simulink model "Pendulum_on_a_Cart"  (R2013b)
settings: Solver=ode3  SolverMode=SingleTasking  StartTime=0.0  StopTime=inf  RelTol=1e-3
values from neighbouring files (symbols this model uses):
  a_b = 0.8    [LEGO_PendulumOnCart_controller.m]    (also in matlab.mat)
  a_d = 0.8    [LEGO_PendulumOnCart_controller.m]    (also in matlab.mat)
  ts1 = 0.004    [LEGO Servo Motor experiments.mat]    (also in LEGO_PendulumOnCart_controller.m; matlab.mat)
  w_n = 172.3/(2*zeta)    (= 86.15)    [LEGO_PendulumOnCart_controller.m]    (also in matlab.mat = 7.59643879413)
  zeta = 1    [LEGO_PendulumOnCart_controller.m]    (also in matlab.mat)
undefined symbols (not defined in the file or in its folder): Kcp, Kv, sigbuilder_block
libraries: legonxtlib x12, simulink x1
settings Model: SimulationMode=external  ExtModeTrigDuration=2  Creator=Alphonso Monk  LastModifiedBy=Alphonso Monk
settings OptimizationCC: OptimizeModelRefInitCode=on  LifeSpan=1
settings DebuggingCC: SolverPrmCheckMsg=none
settings HardwareCC: ProdLargestAtomicInteger=Long  ProdLargestAtomicFloat=Float  ProdEndianess=LittleEndian  ProdHWDeviceType=ARM Compatible->ARM 7
settings RTWCC: SystemTargetFile=realtime.tlc  GenerateMakefile=off  TemplateMakefile=realtime.tmf  Description=Run on Target Hardware  RTWVerbose=off  ProcessScript=realtime_make_rtw_hook
settings STFCustomTargetCC: TargetLibSuffix=.a  GenerateSampleERTMain=on  ERTCustomFileBanners=on  SupportNonInlinedSFcns=off  SupportVariableSizeSignals=on  MATLABClassNameForMDSCustomization=Simulink.SoftwareTarget.ERTCustomization  GRTInterface=off  SystemTargetFile=realtime.tlc
settings ERTTargetCC: CodeReplacementLibrary=ANSI_C  GenerateSampleERTMain=on  ParMdlRefBuildCompliant=off  CompOptLevelCompliant=off  ConcurrentExecutionCompliant=off  CombineOutputUpdateFcns=off  ERTFirstTimeCompliant=off  SupportContinuousTime=on  SupportVariableSizeSignals=on  ModelStepFunctionPrototypeControlCompliant=off  CPPClassGenCompliant=off  ExtMode=on  ExtModeTransport=2  ExtModeMexFile=ext_serial_win32_comm_no_acks_rtt  ExtModeMexArgs=0 3 9600 30  InlinedParameterPlacement=NonHierarchical  ERTSrcFileBannerTemplate=realtime_code_template.cgt  ERTHdrFileBannerTemplate=realtime_code_template.cgt  ERTDataSrcFileTemplate=realtime_code_template.cgt  ERTDataHdrFileTemplate=realtime_code_template.cgt  ERTCustomFileTemplate=realtime_file_process.tlc

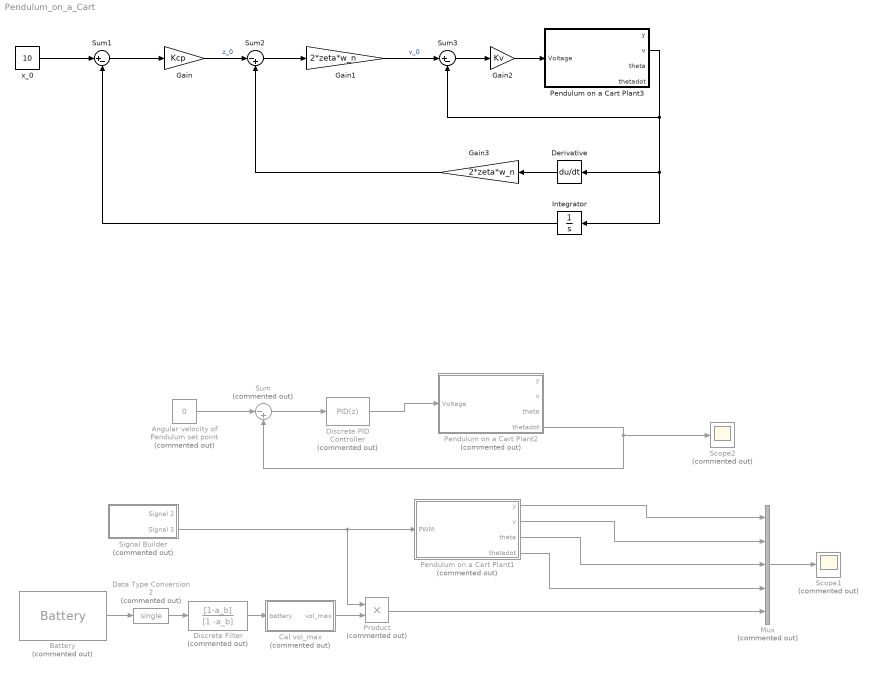
== system Pendulum_on_a_Cart ==
  Angular velocity of Pendulum set point : Constant  Commented=on  Value=0
  Battery : legonxtlib/Battery  Commented=on  sampleTime=ts1
  Cal vol_max : Subsystem  Commented=on
  Data Type Conversion2 : DataTypeConversion  Commented=on  OutDataTypeStr=single  RndMeth=Simplest
  Derivative : Derivative
  Discrete Filter : DiscreteFilter  Commented=on  Numerator=[1-a_b]  Denominator=[1 -a_b]
  Discrete PID Controller : simulink/Continuous/PID Controller  Commented=on  Controller=PID  TimeDomain=Discrete-time  SampleTime=ts1  IntegratorMethod=Forward Euler  FilterMethod=Forward Euler  Form=Parallel  P=0.4059  I=0  D=0  N=100  InitialConditionSource=internal  InitialConditionForIntegrator=0  InitialConditionForFilter=0  ExternalReset=none  LimitOutput=on  UpperSaturationLimit=9  LowerSaturationLimit=-9  LinearizeAsGain=off  AntiWindupMode=none  Kb=1  TrackingMode=off  Kt=1  PParamMin=[]  PParamMax=[]  IParamMin=[]  IParamMax=[]  DParamMin=[]  DParamMax=[]  NParamMin=[]  NParamMax=[]  KbParamMin=[]  KbParamMax=[]  KtParamMin=[]  KtParamMax=[]  POutMin=[]  POutMax=[]  IOutMin=[]  IOutMax=[]  DOutMin=[]  DOutMax=[]  NOutMin=[]  NOutMax=[]  KbOutMin=[]  KbOutMax=[]  KtOutMin=[]  KtOutMax=[]  IntegratorOutMin=[]  IntegratorOutMax=[]  FilterOutMin=[]  FilterOutMax=[]  SumOutMin=[]  SumOutMax=[]  SumI1OutMin=[]  SumI1OutMax=[]  SumI2OutMin=[]  SumI2OutMax=[]  SumI3OutMin=[]  SumI3OutMax=[]  SumDOutMin=[]  SumDOutMax=[]  SaturationOutMin=[]  SaturationOutMax=[]  IntegratorContinuousStateAttributes=''  IntegratorStateMustResolveToSignalObject=off  IntegratorRTWStateStorageClass=Auto  FilterContinuousStateAttributes=''  FilterStateMustResolveToSignalObject=off  FilterRTWStateStorageClass=Auto
  Gain : Gain  Gain=Kcp
  Gain1 : Gain  Gain=2*zeta*w_n
  Gain2 : Gain  Gain=Kv
  Gain3 : Gain  Gain=2*zeta*w_n
  Integrator : Integrator
  Mux : Mux  Commented=on  Inputs=5
  Pendulum on a Cart Plant1 : Subsystem  Commented=on
  Pendulum on a Cart Plant2 : Subsystem  Commented=on
  Pendulum on a Cart Plant3 : Subsystem
  Product : Product  Commented=on
  Scope1 : Scope  Commented=on
      settings: YMin=-600  YMax=600  SaveName=motorResponse1
  Scope2 : Scope  Commented=on
      settings: YMin=1026  YMax=1134  SaveName=motorResponse
  Signal Builder : Subsystem  Tag=STV Subsys  Commented=on  LoadFcn=sigbuilder_block('load');  StartFcn=sigbuilder_block('start');  StopFcn=sigbuilder_block('stop');  ClipboardFcn=sigbuilder_block('clipboard');  mask(Sigbuilder block){}
      mask help: Simulink:masks:SigbuilderBlock_MD
      mask init:
      | if ~strcmp(get_param(bdroot(gcbh),'SimulationStatus'),'stopped') tuvar = sigbuilder_block('maskInit'); end
      settings: CopyFcn=sigbuilder_block('copy');  DeleteFcn=sigbuilder_block('delete');  ModelCloseFcn=sigbuilder_block('modelClose');  PreSaveFcn=sigbuilder_block('preSave');  PauseFcn=sigbuilder_block('pause');  ContinueFcn=sigbuilder_block('continue');  NameChangeFcn=sigbuilder_block('namechange');  OpenFcn=sigbuilder_block('open',[6 28.5 1012.5 484.5 ]);  CloseFcn=sigbuilder_block('close');
      mask Display: plot(0, 0, 100, 100,[2, 2, 32, 32, 2], [68, 8, 8, 68, 68],[32, 2], [38, 38], [32, 19, 2],[53, 60, 44], [32, 17, 17, 2],[16, 16, 31, 31]);txt = getActiveGroup(gcbh);text(2, 100, txt,'verticalAlignment', 'top');
  Sum : Sum  Commented=on  Inputs=|-+
  Sum1 : Sum  Inputs=|+-
  Sum2 : Sum  Inputs=|-+
  Sum3 : Sum  Inputs=|+-
  x_0 : Constant  Value=10
  wires:
  Mux/1 -> Scope1/1
  Signal Builder/2(Signal 3) -> Product/1, Pendulum on a Cart Plant1/1(PWM)
  Product/1 -> Mux/5
  Discrete PID Controller/1 -> Pendulum on a Cart Plant2/1(Voltage)
  Pendulum on a Cart Plant2/4(thetadot) -> Scope2/1, Sum/2
  Sum/1 -> Discrete PID Controller/1
  Angular velocity of Pendulum set point/1 -> Sum/1
  Discrete Filter/1 -> Cal vol_max/1(battery)
  Data Type Conversion2/1 -> Discrete Filter/1
  Battery/1 -> Data Type Conversion2/1
  Cal vol_max/1(vol_max) -> Product/2
  Pendulum on a Cart Plant1/1(y) -> Mux/1
  Pendulum on a Cart Plant1/2(v) -> Mux/2
  Pendulum on a Cart Plant1/3(theta) -> Mux/3
  Pendulum on a Cart Plant1/4(thetadot) -> Mux/4
  x_0/1 -> Sum1/1
  Sum1/1 -> Gain/1
  Gain/1 -> Sum2/1  "z_0"
  Sum2/1 -> Gain1/1
  Gain1/1 -> Sum3/1  "v_0"
  Sum3/1 -> Gain2/1
  Gain2/1 -> Pendulum on a Cart Plant3/1(Voltage)
  Pendulum on a Cart Plant3/2(v) -> Integrator/1, Derivative/1, Sum3/2
  Derivative/1 -> Gain3/1
  Gain3/1 -> Sum2/2
  Integrator/1 -> Sum1/2

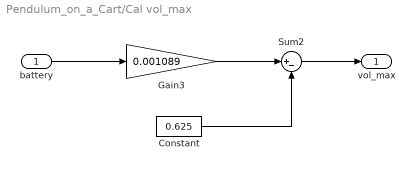
== system Pendulum_on_a_Cart/Cal vol_max ==
  battery : Inport
  Constant : Constant  Value=0.625  OutDataTypeStr=single
      settings: AttributesFormatString=DataType = %<OutDataTypeStr>
  Gain3 : Gain  Gain=0.001089  OutDataTypeStr=Inherit: Same as input  ParamDataTypeStr=Inherit: Same as input
  Sum2 : Sum  Inputs=|+-  OutDataTypeStr=Inherit: Same as first input
  vol_max : Outport
  wires:
  Gain3/1 -> Sum2/1
  Sum2/1 -> vol_max/1
  Constant/1 -> Sum2/2
  battery/1 -> Gain3/1

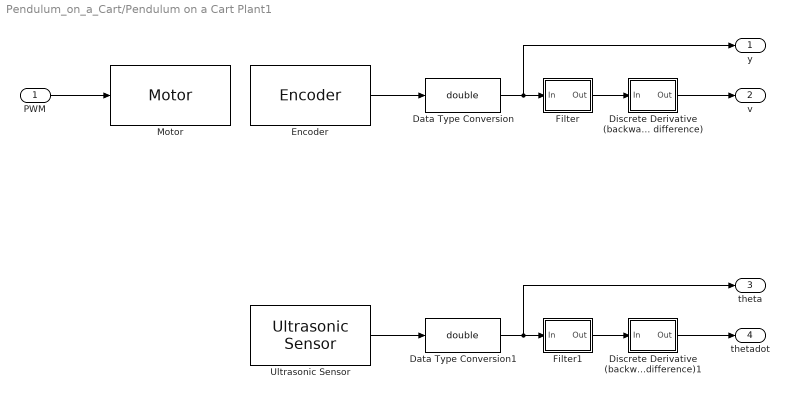
== system Pendulum_on_a_Cart/Pendulum on a Cart Plant1 ==
  PWM : Inport
  Data Type Conversion : DataTypeConversion  OutDataTypeStr=double
  Data Type Conversion1 : DataTypeConversion  OutDataTypeStr=double
  Discrete Derivative (backward difference) : Subsystem
  Discrete Derivative (backward difference)1 : Subsystem
  Encoder : legonxtlib/Encoder  portNumber=B  opMode=No reset  sampleTime=ts1
  Filter : Subsystem
  Filter1 : Subsystem
  Motor : legonxtlib/Motor  sportNumber=B  sstopAction=Brake
  Ultrasonic Sensor : legonxtlib/Ultrasonic Sensor  PortNumber=4  sampleTime=ts1
  y : Outport
  v : Outport  Port=2
  theta : Outport  Port=3
  thetadot : Outport  Port=4
  wires:
  Ultrasonic Sensor/1 -> Data Type Conversion1/1
  Data Type Conversion1/1 -> Filter1/1(In), theta/1
  Filter1/1(Out) -> Discrete Derivative (backward difference)1/1(In)
  Discrete Derivative (backward difference)1/1(Out) -> thetadot/1
  PWM/1 -> Motor/1
  Data Type Conversion/1 -> y/1, Filter/1(In)
  Filter/1(Out) -> Discrete Derivative (backward difference)/1(In)
  Discrete Derivative (backward difference)/1(Out) -> v/1
  Encoder/1 -> Data Type Conversion/1

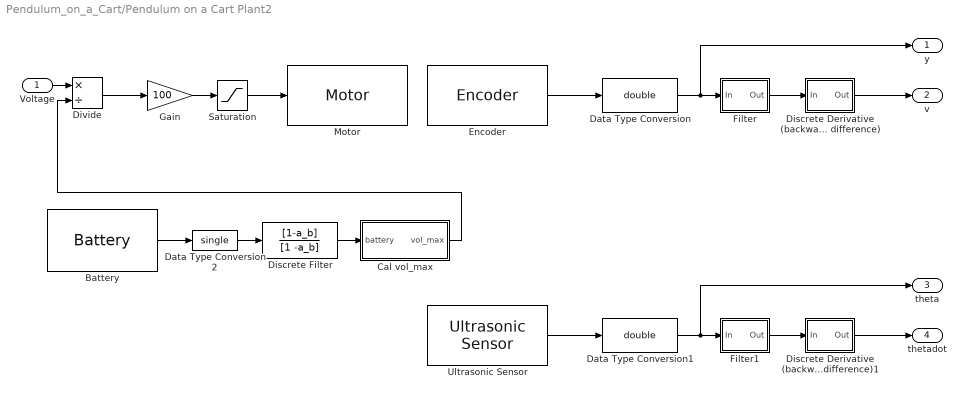
== system Pendulum_on_a_Cart/Pendulum on a Cart Plant2 ==
  Voltage : Inport
  Battery : legonxtlib/Battery  sampleTime=ts1
  Cal vol_max : Subsystem
  Data Type Conversion : DataTypeConversion  OutDataTypeStr=double
  Data Type Conversion1 : DataTypeConversion  OutDataTypeStr=double
  Data Type Conversion2 : DataTypeConversion  OutDataTypeStr=single  RndMeth=Simplest
  Discrete Derivative (backward difference) : Subsystem
  Discrete Derivative (backward difference)1 : Subsystem
  Discrete Filter : DiscreteFilter  Numerator=[1-a_b]  Denominator=[1 -a_b]
  Divide : Product  Inputs=*/
  Encoder : legonxtlib/Encoder  portNumber=B  opMode=No reset  sampleTime=ts1
  Filter : Subsystem
  Filter1 : Subsystem
  Gain : Gain  Gain=100
  Motor : legonxtlib/Motor  sportNumber=B  sstopAction=Brake
  Saturation : Saturate  UpperLimit=100  LowerLimit=-100
  Ultrasonic Sensor : legonxtlib/Ultrasonic Sensor  PortNumber=4  sampleTime=ts1
  y : Outport
  v : Outport  Port=2
  theta : Outport  Port=3
  thetadot : Outport  Port=4
  wires:
  Encoder/1 -> Data Type Conversion/1
  Discrete Derivative (backward difference)/1(Out) -> v/1
  Filter/1(Out) -> Discrete Derivative (backward difference)/1(In)
  Data Type Conversion/1 -> Filter/1(In), y/1
  Gain/1 -> Saturation/1
  Battery/1 -> Data Type Conversion2/1
  Data Type Conversion2/1 -> Discrete Filter/1
  Discrete Filter/1 -> Cal vol_max/1(battery)
  Voltage/1 -> Divide/1
  Cal vol_max/1(vol_max) -> Divide/2
  Divide/1 -> Gain/1
  Saturation/1 -> Motor/1
  Discrete Derivative (backward difference)1/1(Out) -> thetadot/1
  Filter1/1(Out) -> Discrete Derivative (backward difference)1/1(In)
  Data Type Conversion1/1 -> theta/1, Filter1/1(In)
  Ultrasonic Sensor/1 -> Data Type Conversion1/1

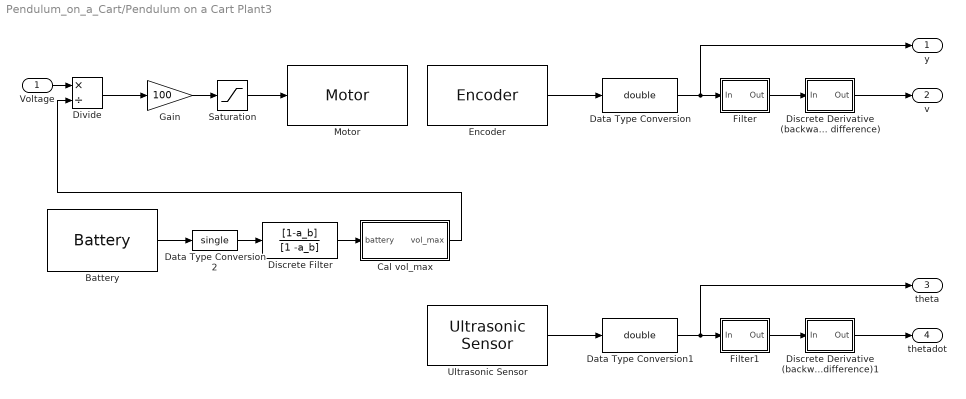
== system Pendulum_on_a_Cart/Pendulum on a Cart Plant3 ==
  Voltage : Inport
  Battery : legonxtlib/Battery  sampleTime=ts1
  Cal vol_max : Subsystem
  Data Type Conversion : DataTypeConversion  OutDataTypeStr=double
  Data Type Conversion1 : DataTypeConversion  OutDataTypeStr=double
  Data Type Conversion2 : DataTypeConversion  OutDataTypeStr=single  RndMeth=Simplest
  Discrete Derivative (backward difference) : Subsystem
  Discrete Derivative (backward difference)1 : Subsystem
  Discrete Filter : DiscreteFilter  Numerator=[1-a_b]  Denominator=[1 -a_b]
  Divide : Product  Inputs=*/
  Encoder : legonxtlib/Encoder  portNumber=B  opMode=No reset  sampleTime=ts1
  Filter : Subsystem
  Filter1 : Subsystem
  Gain : Gain  Gain=100
  Motor : legonxtlib/Motor  sportNumber=B  sstopAction=Brake
  Saturation : Saturate  UpperLimit=100  LowerLimit=-100
  Ultrasonic Sensor : legonxtlib/Ultrasonic Sensor  PortNumber=4  sampleTime=ts1
  y : Outport
  v : Outport  Port=2
  theta : Outport  Port=3
  thetadot : Outport  Port=4
  wires:
  Ultrasonic Sensor/1 -> Data Type Conversion1/1
  Data Type Conversion1/1 -> Filter1/1(In), theta/1
  Filter1/1(Out) -> Discrete Derivative (backward difference)1/1(In)
  Discrete Derivative (backward difference)1/1(Out) -> thetadot/1
  Saturation/1 -> Motor/1
  Divide/1 -> Gain/1
  Cal vol_max/1(vol_max) -> Divide/2
  Voltage/1 -> Divide/1
  Discrete Filter/1 -> Cal vol_max/1(battery)
  Data Type Conversion2/1 -> Discrete Filter/1
  Battery/1 -> Data Type Conversion2/1
  Gain/1 -> Saturation/1
  Data Type Conversion/1 -> y/1, Filter/1(In)
  Filter/1(Out) -> Discrete Derivative (backward difference)/1(In)
  Discrete Derivative (backward difference)/1(Out) -> v/1
  Encoder/1 -> Data Type Conversion/1

== system Pendulum_on_a_Cart/Signal Builder ==
  Demux : Demux  Tag=STV Demux  Outputs=2
  FromWs : FromWorkspace  Tag=STV FromWs  VariableName=tuvar  SampleTime=0
      SigBuilderData=|
      | common.afterFinalStr = 'Extrapolate'
      | common.sampleTime = 0
      | dataSet.timeRange = [0 30]
      | dataSet.name = 'Group 1'
      | sbobj.Groups.Name = 'Group 1'
      | sbobj.Groups.Signals(1).Name = 'Signal 2'
      | sbobj.Groups.Signals(1).XData = [0 3 3 7 7 30]
      | sbobj.Groups.Signals(1).YData = [0 0 100 100 0 0]
      | sbobj.Groups.Signals(2).Name = 'Signal 3'
      | sbobj.Groups.Signals(2).XData = [0 1 1 1.5 1.5 2.5 2.5 3.5 3.5 5 5 5.5 5.5 6.5 6.5 7 7 7.5 7.5 8.5 8.5 10.5 10.5 11 11 13.5 13.5 14 14 14.5 14.5 15 15 15.5 15.5 17.5 17.5 18.5 18.5 19 19 19.5 19.5 21 21 22 22 23.5 23.5 25 25 25.5 25.5 26.5 26.5 28 28 28.5 28.5 29 29 29.5 29.5 30]
      | sbobj.Groups.Signals(2).YData = [100 100 -100 -100 100 100 -100 -100 100 100 -100 -100 100 100 -100 -100 100 100 -100 -100 100 100 -100 -100 100 100 -100 -100 100 100 -100 -100 100 100 -100 -100 100 100 -100 -100 100 100 -100 -100 100 100 -100 -100 100 100 -100 -100 100 100 -100 -100 100 100 -100 -100 100 100 -100 -100]
      | sbobj.Groups.TimeRange = [0 30]
  Signal 2 : Outport  Tag=STV Outport
  Signal 3 : Outport  Tag=STV Outport  Port=2
  wires:
  FromWs/1 -> Demux/1
  Demux/1 -> Signal 2/1
  Demux/2 -> Signal 3/1

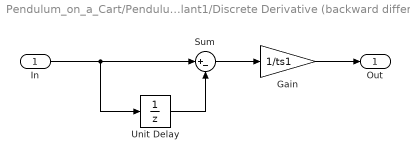
== system Pendulum_on_a_Cart/Pendulum on a Cart Plant1/Discrete Derivative (backward difference) ==
  In : Inport
  Gain : Gain  Gain=1/ts1  OutDataTypeStr=Inherit: Same as input  ParamDataTypeStr=Inherit: Same as input
  Sum : Sum  Inputs=|+-  OutDataTypeStr=Inherit: Same as first input
  Unit Delay : UnitDelay  SampleTime=-1
  Out : Outport
  wires:
  Sum/1 -> Gain/1
  Unit Delay/1 -> Sum/2
  In/1 -> Unit Delay/1, Sum/1
  Gain/1 -> Out/1

== system Pendulum_on_a_Cart/Pendulum on a Cart Plant1/Discrete Derivative (backward difference)1 ==
  In : Inport
  Gain : Gain  Gain=1/ts1  OutDataTypeStr=Inherit: Same as input  ParamDataTypeStr=Inherit: Same as input
  Sum : Sum  Inputs=|+-  OutDataTypeStr=Inherit: Same as first input
  Unit Delay : UnitDelay  SampleTime=-1
  Out : Outport
  wires:
  Gain/1 -> Out/1
  In/1 -> Sum/1, Unit Delay/1
  Unit Delay/1 -> Sum/2
  Sum/1 -> Gain/1

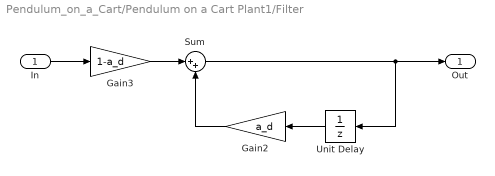
== system Pendulum_on_a_Cart/Pendulum on a Cart Plant1/Filter ==
  In : Inport
  Gain2 : Gain  Gain=a_d  OutDataTypeStr=Inherit: Same as input  ParamDataTypeStr=Inherit: Same as input
  Gain3 : Gain  Gain=1-a_d  OutDataTypeStr=Inherit: Same as input  ParamDataTypeStr=Inherit: Same as input
  Sum : Sum  Inputs=|++  OutDataTypeStr=Inherit: Same as first input
  Unit Delay : UnitDelay  SampleTime=-1
  Out : Outport
  wires:
  Sum/1 -> Unit Delay/1, Out/1
  Unit Delay/1 -> Gain2/1
  Gain2/1 -> Sum/2
  Gain3/1 -> Sum/1
  In/1 -> Gain3/1

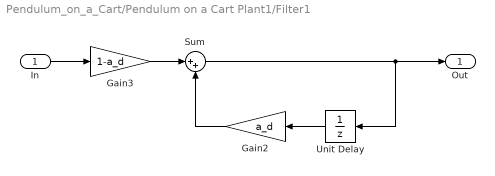
== system Pendulum_on_a_Cart/Pendulum on a Cart Plant1/Filter1 ==
  In : Inport
  Gain2 : Gain  Gain=a_d  OutDataTypeStr=Inherit: Same as input  ParamDataTypeStr=Inherit: Same as input
  Gain3 : Gain  Gain=1-a_d  OutDataTypeStr=Inherit: Same as input  ParamDataTypeStr=Inherit: Same as input
  Sum : Sum  Inputs=|++  OutDataTypeStr=Inherit: Same as first input
  Unit Delay : UnitDelay  SampleTime=-1
  Out : Outport
  wires:
  In/1 -> Gain3/1
  Gain3/1 -> Sum/1
  Gain2/1 -> Sum/2
  Unit Delay/1 -> Gain2/1
  Sum/1 -> Out/1, Unit Delay/1

== system Pendulum_on_a_Cart/Pendulum on a Cart Plant2/Cal vol_max ==
  battery : Inport
  Constant : Constant  Value=0.625  OutDataTypeStr=single
      settings: AttributesFormatString=DataType = %<OutDataTypeStr>
  Gain3 : Gain  Gain=0.001089  OutDataTypeStr=Inherit: Same as input  ParamDataTypeStr=Inherit: Same as input
  Sum2 : Sum  Inputs=|+-  OutDataTypeStr=Inherit: Same as first input
  vol_max : Outport
  wires:
  battery/1 -> Gain3/1
  Constant/1 -> Sum2/2
  Sum2/1 -> vol_max/1
  Gain3/1 -> Sum2/1

== system Pendulum_on_a_Cart/Pendulum on a Cart Plant2/Discrete Derivative (backward difference) ==
  In : Inport
  Gain : Gain  Gain=1/ts1  OutDataTypeStr=Inherit: Same as input  ParamDataTypeStr=Inherit: Same as input
  Sum : Sum  Inputs=|+-  OutDataTypeStr=Inherit: Same as first input
  Unit Delay : UnitDelay  SampleTime=-1
  Out : Outport
  wires:
  Gain/1 -> Out/1
  In/1 -> Sum/1, Unit Delay/1
  Unit Delay/1 -> Sum/2
  Sum/1 -> Gain/1

== system Pendulum_on_a_Cart/Pendulum on a Cart Plant2/Discrete Derivative (backward difference)1 ==
  In : Inport
  Gain : Gain  Gain=1/ts1  OutDataTypeStr=Inherit: Same as input  ParamDataTypeStr=Inherit: Same as input
  Sum : Sum  Inputs=|+-  OutDataTypeStr=Inherit: Same as first input
  Unit Delay : UnitDelay  SampleTime=-1
  Out : Outport
  wires:
  Sum/1 -> Gain/1
  Unit Delay/1 -> Sum/2
  In/1 -> Unit Delay/1, Sum/1
  Gain/1 -> Out/1

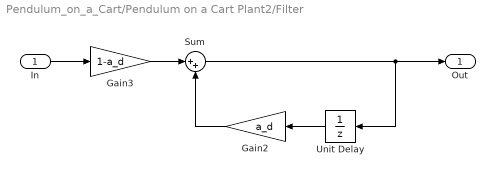
== system Pendulum_on_a_Cart/Pendulum on a Cart Plant2/Filter ==
  In : Inport
  Gain2 : Gain  Gain=a_d  OutDataTypeStr=Inherit: Same as input  ParamDataTypeStr=Inherit: Same as input
  Gain3 : Gain  Gain=1-a_d  OutDataTypeStr=Inherit: Same as input  ParamDataTypeStr=Inherit: Same as input
  Sum : Sum  Inputs=|++  OutDataTypeStr=Inherit: Same as first input
  Unit Delay : UnitDelay  SampleTime=-1
  Out : Outport
  wires:
  In/1 -> Gain3/1
  Gain3/1 -> Sum/1
  Gain2/1 -> Sum/2
  Unit Delay/1 -> Gain2/1
  Sum/1 -> Out/1, Unit Delay/1

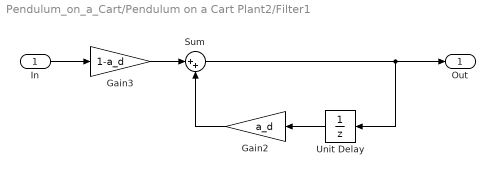
== system Pendulum_on_a_Cart/Pendulum on a Cart Plant2/Filter1 ==
  In : Inport
  Gain2 : Gain  Gain=a_d  OutDataTypeStr=Inherit: Same as input  ParamDataTypeStr=Inherit: Same as input
  Gain3 : Gain  Gain=1-a_d  OutDataTypeStr=Inherit: Same as input  ParamDataTypeStr=Inherit: Same as input
  Sum : Sum  Inputs=|++  OutDataTypeStr=Inherit: Same as first input
  Unit Delay : UnitDelay  SampleTime=-1
  Out : Outport
  wires:
  Sum/1 -> Unit Delay/1, Out/1
  Unit Delay/1 -> Gain2/1
  Gain2/1 -> Sum/2
  Gain3/1 -> Sum/1
  In/1 -> Gain3/1

== system Pendulum_on_a_Cart/Pendulum on a Cart Plant3/Cal vol_max ==
  battery : Inport
  Constant : Constant  Value=0.625  OutDataTypeStr=single
      settings: AttributesFormatString=DataType = %<OutDataTypeStr>
  Gain3 : Gain  Gain=0.001089  OutDataTypeStr=Inherit: Same as input  ParamDataTypeStr=Inherit: Same as input
  Sum2 : Sum  Inputs=|+-  OutDataTypeStr=Inherit: Same as first input
  vol_max : Outport
  wires:
  Gain3/1 -> Sum2/1
  Sum2/1 -> vol_max/1
  Constant/1 -> Sum2/2
  battery/1 -> Gain3/1

== system Pendulum_on_a_Cart/Pendulum on a Cart Plant3/Discrete Derivative (backward difference) ==
  In : Inport
  Gain : Gain  Gain=1/ts1  OutDataTypeStr=Inherit: Same as input  ParamDataTypeStr=Inherit: Same as input
  Sum : Sum  Inputs=|+-  OutDataTypeStr=Inherit: Same as first input
  Unit Delay : UnitDelay  SampleTime=-1
  Out : Outport
  wires:
  Sum/1 -> Gain/1
  Unit Delay/1 -> Sum/2
  In/1 -> Unit Delay/1, Sum/1
  Gain/1 -> Out/1

== system Pendulum_on_a_Cart/Pendulum on a Cart Plant3/Discrete Derivative (backward difference)1 ==
  In : Inport
  Gain : Gain  Gain=1/ts1  OutDataTypeStr=Inherit: Same as input  ParamDataTypeStr=Inherit: Same as input
  Sum : Sum  Inputs=|+-  OutDataTypeStr=Inherit: Same as first input
  Unit Delay : UnitDelay  SampleTime=-1
  Out : Outport
  wires:
  Gain/1 -> Out/1
  In/1 -> Sum/1, Unit Delay/1
  Unit Delay/1 -> Sum/2
  Sum/1 -> Gain/1

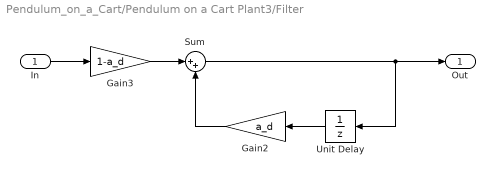
== system Pendulum_on_a_Cart/Pendulum on a Cart Plant3/Filter ==
  In : Inport
  Gain2 : Gain  Gain=a_d  OutDataTypeStr=Inherit: Same as input  ParamDataTypeStr=Inherit: Same as input
  Gain3 : Gain  Gain=1-a_d  OutDataTypeStr=Inherit: Same as input  ParamDataTypeStr=Inherit: Same as input
  Sum : Sum  Inputs=|++  OutDataTypeStr=Inherit: Same as first input
  Unit Delay : UnitDelay  SampleTime=-1
  Out : Outport
  wires:
  Sum/1 -> Unit Delay/1, Out/1
  Unit Delay/1 -> Gain2/1
  Gain2/1 -> Sum/2
  Gain3/1 -> Sum/1
  In/1 -> Gain3/1

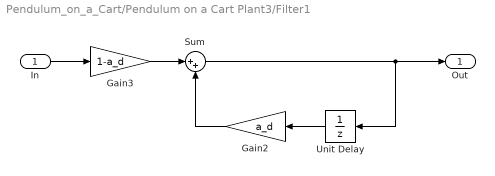
== system Pendulum_on_a_Cart/Pendulum on a Cart Plant3/Filter1 ==
  In : Inport
  Gain2 : Gain  Gain=a_d  OutDataTypeStr=Inherit: Same as input  ParamDataTypeStr=Inherit: Same as input
  Gain3 : Gain  Gain=1-a_d  OutDataTypeStr=Inherit: Same as input  ParamDataTypeStr=Inherit: Same as input
  Sum : Sum  Inputs=|++  OutDataTypeStr=Inherit: Same as first input
  Unit Delay : UnitDelay  SampleTime=-1
  Out : Outport
  wires:
  In/1 -> Gain3/1
  Gain3/1 -> Sum/1
  Gain2/1 -> Sum/2
  Unit Delay/1 -> Gain2/1
  Sum/1 -> Out/1, Unit Delay/1
